simulink model "modele_simplifie_simulink2024"  (R2024a)
settings: Solver=VariableStepAuto  StartTime=0.0  StopTime=T_att  RelTol=1e-3
values from neighbouring files (symbols this model uses):
  g = 9.81    [script_devoir2.m]
  isQ3a = false    [script_devoir2.m]
  Kdx = -0.367    [script_devoir2.m]
  Kdy = 15000    [script_devoir2.m]
  Kix = -0.176    [script_devoir2.m]
  Kiy = 125000    [script_devoir2.m]
  Kpx = -0.440    (= -0.44)    [script_devoir2.m]
  Kpy = 75000    [script_devoir2.m]
  m = 1000    [script_devoir2.m]
  x0 = [x0_pos; vx0; y0_pos; vy0; 0; 0]    [script_devoir2.m]
settings Model: Creator=andreagourion  LastModifiedBy=Andrea
settings ConfigComp: CovBoundaryAbsTol=1.0e-5

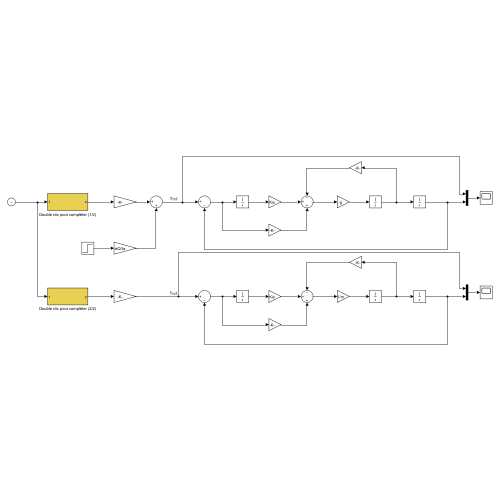
[thumbnail: Simulink's stored preview of the top-level diagram]
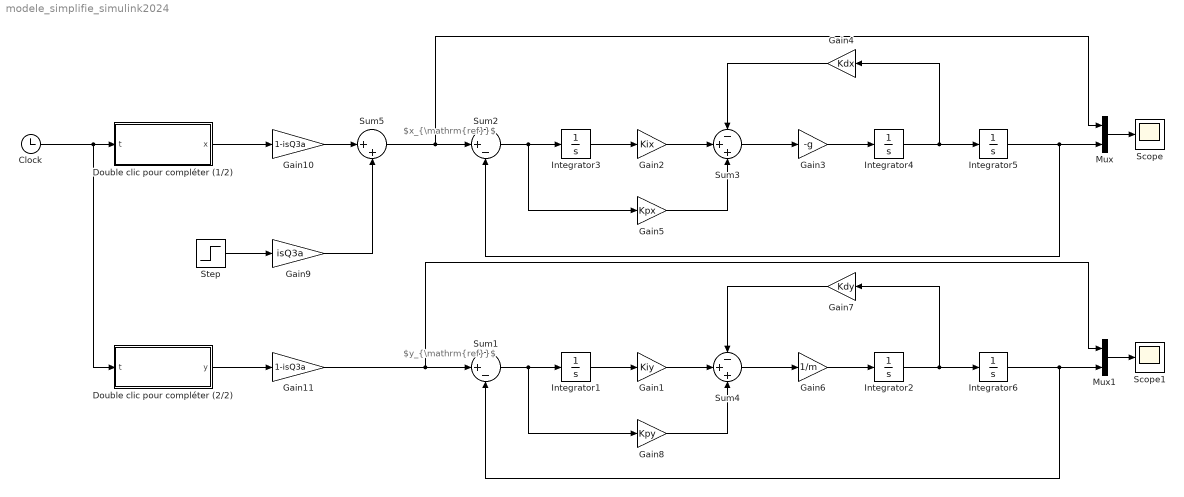
== system modele_simplifie_simulink2024 ==
  note: $x_{\mathrm{ref}}$
  note: $y_{\mathrm{ref}}$
  Clock : Clock
  Double clic pour compléter (1/2) : Subsystem
  Double clic pour compléter (2/2) : Subsystem
  Gain1 : Gain  Gain=Kiy
  Gain10 : Gain  Gain=1-isQ3a
  Gain11 : Gain  Gain=1-isQ3a
  Gain2 : Gain  Gain=Kix
  Gain3 : Gain  Gain=-g
  Gain4 : Gain  Gain=Kdx
  Gain5 : Gain  Gain=Kpx
  Gain6 : Gain  Gain=1/m
  Gain7 : Gain  Gain=Kdy
  Gain8 : Gain  Gain=Kpy
  Gain9 : Gain  Gain=isQ3a
  Integrator1 : Integrator
  Integrator2 : Integrator  InitialCondition=x0(4)
  Integrator3 : Integrator
  Integrator4 : Integrator  InitialCondition=x0(2)
  Integrator5 : Integrator  InitialCondition=x0(1)
  Integrator6 : Integrator  InitialCondition=x0(3)
  Mux : Mux  Inputs=2
  Mux1 : Mux  Inputs=2
  Scope : Scope
  Scope1 : Scope
  Step : Step  Time=0  SampleTime=0
  Sum1 : Sum  Inputs=|+-
  Sum2 : Sum  Inputs=|+-
  Sum3 : Sum  Inputs=-++
  Sum4 : Sum  Inputs=-++
  Sum5 : Sum  Inputs=|++
  wires:
  Clock/1 -> Double clic pour compléter (1/2)/1(t), Double clic pour compléter (2/2)/1(t)
  Integrator3/1 -> Gain2/1
  Sum2/1 -> Gain5/1, Integrator3/1
  Integrator4/1 -> Gain4/1, Integrator5/1
  Gain2/1 -> Sum3/2
  Sum3/1 -> Gain3/1
  Gain3/1 -> Integrator4/1
  Gain4/1 -> Sum3/1
  Gain5/1 -> Sum3/3
  Integrator5/1 -> Mux/2, Sum2/2
  Sum1/1 -> Gain8/1, Integrator1/1
  Sum4/1 -> Gain6/1
  Integrator1/1 -> Gain1/1
  Gain6/1 -> Integrator2/1
  Integrator2/1 -> Gain7/1, Integrator6/1
  Gain1/1 -> Sum4/2
  Gain7/1 -> Sum4/1
  Gain8/1 -> Sum4/3
  Mux/1 -> Scope/1
  Mux1/1 -> Scope1/1
  Integrator6/1 -> Sum1/2, Mux1/2
  Double clic pour compléter (2/2)/1(y) -> Gain11/1
  Step/1 -> Gain9/1
  Double clic pour compléter (1/2)/1(x) -> Gain10/1
  Sum5/1 -> Mux/1, Sum2/1
  Gain9/1 -> Sum5/2
  Gain10/1 -> Sum5/1
  Gain11/1 -> Mux1/1, Sum1/1

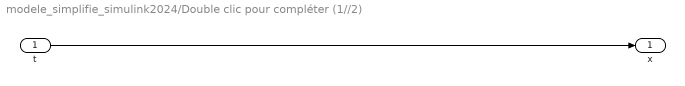
== system modele_simplifie_simulink2024/Double clic pour compléter (1//2) ==
  t : Inport
  x : Outport
  wires:
  t/1 -> x/1

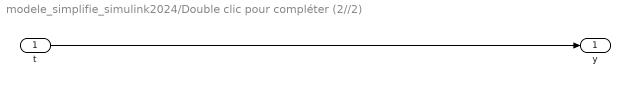
== system modele_simplifie_simulink2024/Double clic pour compléter (2//2) ==
  t : Inport
  y : Outport
  wires:
  t/1 -> y/1
